simulink model "TP1"  (R2023a)
settings: Solver=VariableStepAuto  StartTime=0.0  StopTime=5  RelTol=1e-9  AbsTol=1e-9
values from neighbouring files (symbols this model uses):
  Beff = 1/80    (= 0.0125)    [sf_loi_avant_RP.m]    (also in sf_retour_linearisant_boucle_interne_RP.m; valeurs.m)
  Jeff = Jm + (r^2)*m    (= 0.010375)    [sf_loi_avant_RP.m]    (also in sf_retour_linearisant_boucle_interne_RP.m = 15.01; valeurs.m = 15.01)
  K = (4*Jeff)/((e.^2)*(KR))    [sf_loi_avant_RP.m]    (also in sf_retour_linearisant_boucle_interne_RP.m; valeurs.m)
  Kd = ((4*Jeff)/(1/2) - Beff)/KR    (= 0.235)    [sf_loi_avant_RP.m]    (also in sf_retour_linearisant_boucle_interne_RP.m = 400.225; valeurs.m = 400.225)
  KR = 0.3    [sf_loi_avant_RP.m]    (also in sf_retour_linearisant_boucle_interne_RP.m; valeurs.m)
  r = 1/200    (= 0.005)    [sf_loi_avant_RP.m]    (also in sf_retour_linearisant_boucle_interne_RP.m = 1; valeurs.m = 1)
libraries: simulink x1
settings Model: Creator=GWC4238A  LastModifiedBy=GWC4238A

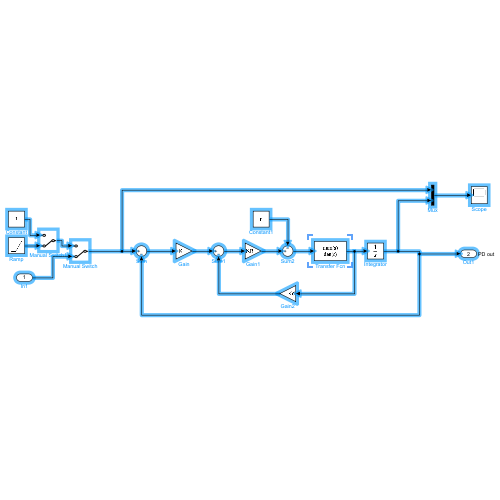
[thumbnail: Simulink's stored preview of the top-level diagram]
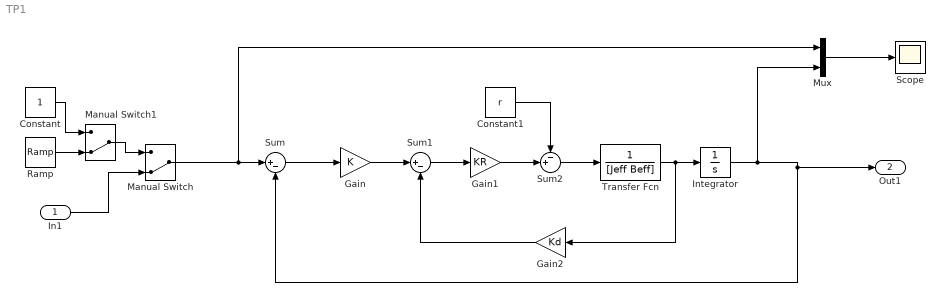
== system TP1 ==
  In1 : Inport
  Constant : Constant
  Constant1 : Constant  Value=r
  Gain : Gain  Gain=K
  Gain1 : Gain  Gain=KR
  Gain2 : Gain  Gain=Kd
  Integrator : Integrator
  Manual Switch : ManualSwitch  CurrentSetting=0
  Manual Switch1 : ManualSwitch  CurrentSetting=0
  Mux : Mux  Inputs=2
  Ramp : simulink/Sources/Ramp  slope=1  start=0  InitialOutput=0
  Scope : Scope
  Sum : Sum  Inputs=|+-
  Sum1 : Sum  Inputs=|+-
  Sum2 : Sum  Inputs=-+|
  Transfer Fcn : TransferFcn  Denominator=[Jeff Beff]
  Out1 : Outport  Port=2  SignalName=PD out
  wires:
  Sum/1 -> Gain/1
  Gain/1 -> Sum1/1
  Sum1/1 -> Gain1/1
  Gain1/1 -> Sum2/2
  Sum2/1 -> Transfer Fcn/1
  Transfer Fcn/1 -> Gain2/1, Integrator/1
  Gain2/1 -> Sum1/2
  Integrator/1 -> Sum/2, Out1/1, Mux/2
  Manual Switch/1 -> Mux/1, Sum/1
  Mux/1 -> Scope/1
  Constant1/1 -> Sum2/1
  Manual Switch1/1 -> Manual Switch/1
  Constant/1 -> Manual Switch1/1
  Ramp/1 -> Manual Switch1/2
  In1/1 -> Manual Switch/2
